simulink library "dlbsBlockRelu"  (R2025b)
settings: Solver=VariableStepAuto  StartTime=0.0  StopTime=10.0  RelTol=1e-3
libraries: simulink x1, dlbsBlockExtractGradientGF x1, dlbsBlockInsertGradientGF x1
settings Model: Creator=lt6037  LastModifiedBy=lt6037

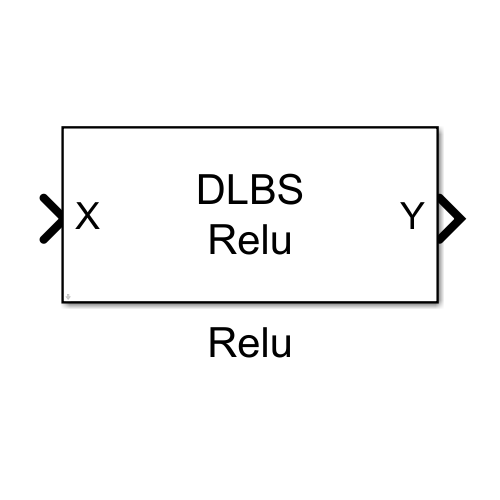
[thumbnail: Simulink's stored preview of the top-level diagram]
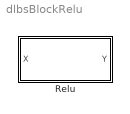
== system dlbsBlockRelu ==
  Relu : Subsystem
      mask help: Applies the rectified linear unit activation to the input tensor. The operation is applied element-wise across all tensor elements.
      mask Help: web("dlbsHelpBlockRelu.html")
      mask Display: fprintf("DLBS\nRelu")

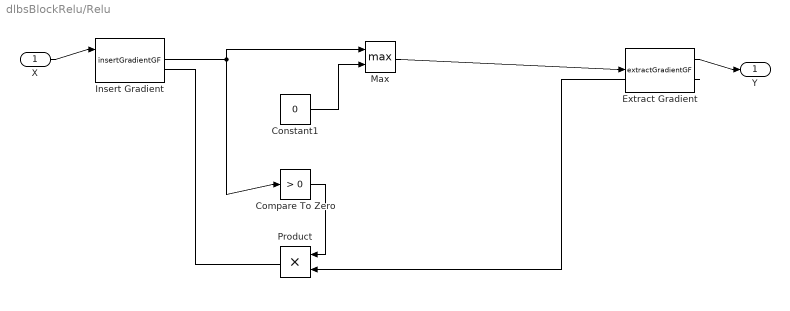
== system dlbsBlockRelu/Relu ==
  X : Inport
  Compare To Zero : simulink/Logic and Bit Operations/Compare To Zero  relop=>  OutDataTypeStr=boolean
  Constant1 : Constant  Value=0  OutDataTypeStr=Inherit: Inherit via back propagation
  Extract Gradient : dlbsBlockExtractGradientGF/extractGradientGF
  Insert Gradient : dlbsBlockInsertGradientGF/insertGradientGF
  Max : MinMax  Function=max  Inputs=2
  Product : Product
  Y : Outport
  wires:
  Insert Gradient/1 -> Compare To Zero/1, Max/1
  Max/1 -> Extract Gradient/1
  Constant1/1 -> Max/2
  Compare To Zero/1 -> Product/1
  Extract Gradient/2 -> Product/2
  Product/1 -> Insert Gradient/2
  Extract Gradient/1 -> Y/1
  X/1 -> Insert Gradient/1
